simulink model "aerotest"  (R2021b)
settings: Solver=VariableStepAuto  StartTime=0.0  StopTime=10.0  RelTol=1e-3
undefined symbols (not defined in the file or in its folder): admireDB
libraries: simulink_extras x103, simulink x24, aerolibatmos2 x1
(part 9 of 13)

== system aerotest/CentripetalForceCoefficient/MachRegion4/Ccblg/Ccblg_ ==
  ldg : Inport
  angleOfAttack_deg : Inport  Port=2
  angleOfSideslip_deg : Inport  Port=3
  CCBLST_NG_DOOR_ALFA : Lookup_n-D  BreakpointsForDimension1=admireDB.aerodata_asym_ext.CCBLST.breakpoints.ALFA  BreakpointsForDimension2=admireDB.aerodata_asym_ext.CCBLST.breakpoints.NG_DOOR  BreakpointsForDimension3=[5, 7]  Table=admireDB.aerodata_asym_ext.CCBLST.newTable  ExtrapMethod=Clip  InternalRulePriority=Speed  RndMeth=Simplest  InputSameDT=on
      settings: InputPortMap=u0,u1
  Degrees to Radians : simulink_extras/Transformations/Degrees to Radians
  Product : Product  Inputs=3
  Ccblg : Outport
  wires:
  Degrees to Radians/1 -> Product/3
  CCBLST_NG_DOOR_ALFA/1 -> Product/2
  angleOfSideslip_deg/1 -> Degrees to Radians/1
  ldg/1 -> CCBLST_NG_DOOR_ALFA/2, Product/1
  angleOfAttack_deg/1 -> CCBLST_NG_DOOR_ALFA/1
  Product/1 -> Ccblg/1

== system aerotest/CentripetalForceCoefficient/MachRegion4/Ccdai/Ccdai_ ==
  dAI : Inport
  angleOfAttack_deg : Inport  Port=2
  dEI : Inport  Port=3
  qacorr : Inport  Port=4
  eieff : Inport  Port=5
  mach_nd : Inport  Port=6
  CCDA_ALFA_DE_M : Lookup_n-D  NumberOfTableDimensions=3  BreakpointsForDimension1=admireDB.aerodata_asym_ext.CCDA.breakpoints.ALFA  BreakpointsForDimension2=admireDB.aerodata_asym_ext.CCDA.breakpoints.DE  BreakpointsForDimension3=admireDB.aerodata_asym_ext.CCDA.breakpoints.M  Table=admireDB.aerodata_asym_ext.CCDA.newTable  ExtrapMethod=Clip  InternalRulePriority=Speed  RndMeth=Simplest  InputSameDT=on
      settings: InputPortMap=u0,u1,u2
  CCEDAI_QA_M : Lookup_n-D  BreakpointsForDimension1=admireDB.aerodata_asym_ext.CCEDAI.breakpoints.M  BreakpointsForDimension2=admireDB.aerodata_asym_ext.CCEDAI.breakpoints.QA  BreakpointsForDimension3=[5, 7]  Table=admireDB.aerodata_asym_ext.CCEDAI.newTable  ExtrapMethod=Clip  InternalRulePriority=Speed  RndMeth=Simplest  InputSameDT=on
      settings: InputPortMap=u0,u1
  Degrees to Radians : simulink_extras/Transformations/Degrees to Radians
  Product1 : Product  Inputs=4
  Ccdai : Outport
  wires:
  Product1/1 -> Ccdai/1
  eieff/1 -> Product1/2
  CCEDAI_QA_M/1 -> Product1/4
  qacorr/1 -> CCEDAI_QA_M/2
  dEI/1 -> CCDA_ALFA_DE_M/2
  CCDA_ALFA_DE_M/1 -> Product1/3
  Degrees to Radians/1 -> Product1/1
  mach_nd/1 -> CCDA_ALFA_DE_M/3, CCEDAI_QA_M/1
  angleOfAttack_deg/1 -> CCDA_ALFA_DE_M/1
  dAI/1 -> Degrees to Radians/1

== system aerotest/CentripetalForceCoefficient/MachRegion4/Ccday/Ccday_ ==
  angleOfAttack_deg : Inport
  dEY : Inport  Port=2
  mach_nd : Inport  Port=3
  qacorr : Inport  Port=4
  eoeff : Inport  Port=5
  dAY : Inport  Port=6
  CCDA_ALFA_DE_M : Lookup_n-D  NumberOfTableDimensions=3  BreakpointsForDimension1=admireDB.aerodata_asym_ext.CCDA.breakpoints.ALFA  BreakpointsForDimension2=admireDB.aerodata_asym_ext.CCDA.breakpoints.DE  BreakpointsForDimension3=admireDB.aerodata_asym_ext.CCDA.breakpoints.M  Table=admireDB.aerodata_asym_ext.CCDA.newTable  ExtrapMethod=Clip  InternalRulePriority=Speed  RndMeth=Simplest  InputSameDT=on
      settings: InputPortMap=u0,u1,u2
  CCEDAY_QA_M : Lookup_n-D  BreakpointsForDimension1=admireDB.aerodata_asym_ext.CCEDAY.breakpoints.M  BreakpointsForDimension2=admireDB.aerodata_asym_ext.CCEDAY.breakpoints.QA  BreakpointsForDimension3=[5, 7]  Table=admireDB.aerodata_asym_ext.CCEDAY.newTable  ExtrapMethod=Clip  InternalRulePriority=Speed  RndMeth=Simplest  InputSameDT=on
      settings: InputPortMap=u0,u1
  Degrees to Radians : simulink_extras/Transformations/Degrees to Radians
  Product : Product
  Product1 : Product
  Sum : Sum  Inputs=|++
  Ccday : Outport
  wires:
  Product1/1 -> Ccday/1
  dAY/1 -> Degrees to Radians/1
  Degrees to Radians/1 -> Product1/2
  Sum/1 -> Product1/1
  qacorr/1 -> CCEDAY_QA_M/2
  CCEDAY_QA_M/1 -> Sum/2
  Product/1 -> Sum/1
  CCDA_ALFA_DE_M/1 -> Product/1
  eoeff/1 -> Product/2
  mach_nd/1 -> CCDA_ALFA_DE_M/3, CCEDAY_QA_M/1
  dEY/1 -> CCDA_ALFA_DE_M/2
  angleOfAttack_deg/1 -> CCDA_ALFA_DE_M/1

== system aerotest/CentripetalForceCoefficient/MachRegion4/Ccdna/Ccdna_ ==
  angleOfAttack_deg : Inport
  mach_nd : Inport  Port=2
  dNA : Inport  Port=3
  CCDNAAM_ALFA_M : Lookup_n-D  BreakpointsForDimension1=admireDB.aerodata_asym_ext.CCDNAAM.breakpoints.M  BreakpointsForDimension2=admireDB.aerodata_asym_ext.CCDNAAM.breakpoints.ALFA  BreakpointsForDimension3=[5, 7]  Table=admireDB.aerodata_asym_ext.CCDNAAM.newTable  ExtrapMethod=Clip  InternalRulePriority=Speed  RndMeth=Simplest  InputSameDT=on
      settings: InputPortMap=u0,u1
  Degrees to Radians : simulink_extras/Transformations/Degrees to Radians
  Product1 : Product
  Ccdna : Outport
  wires:
  Degrees to Radians/1 -> Product1/2
  dNA/1 -> Degrees to Radians/1
  Product1/1 -> Ccdna/1
  mach_nd/1 -> CCDNAAM_ALFA_M/1
  CCDNAAM_ALFA_M/1 -> Product1/1
  angleOfAttack_deg/1 -> CCDNAAM_ALFA_M/2

== system aerotest/CentripetalForceCoefficient/MachRegion4/Ccdr/Ccdr_ ==
  angleOfAttack_deg : Inport
  mach_nd : Inport  Port=2
  dR : Inport  Port=3
  qacorr : Inport  Port=4
  CCDRAM_ALFA_M : Lookup_n-D  BreakpointsForDimension1=admireDB.aerodata_asym_ext.CCDRAM.breakpoints.M  BreakpointsForDimension2=admireDB.aerodata_asym_ext.CCDRAM.breakpoints.ALFA  BreakpointsForDimension3=[5, 7]  Table=admireDB.aerodata_asym_ext.CCDRAM.newTable  ExtrapMethod=Clip  InternalRulePriority=Speed  RndMeth=Simplest  InputSameDT=on
      settings: InputPortMap=u0,u1
  CCEDR_QA_M : Lookup_n-D  BreakpointsForDimension1=admireDB.aerodata_asym_ext.CCEDR.breakpoints.M  BreakpointsForDimension2=admireDB.aerodata_asym_ext.CCEDR.breakpoints.QA  BreakpointsForDimension3=[5, 7]  Table=admireDB.aerodata_asym_ext.CCEDR.newTable  ExtrapMethod=Clip  InternalRulePriority=Speed  RndMeth=Simplest  InputSameDT=on
      settings: InputPortMap=u0,u1
  Degrees to Radians : simulink_extras/Transformations/Degrees to Radians
  Product1 : Product  Inputs=3
  Ccdr : Outport
  wires:
  CCEDR_QA_M/1 -> Product1/3
  Product1/1 -> Ccdr/1
  mach_nd/1 -> CCEDR_QA_M/1, CCDRAM_ALFA_M/1
  qacorr/1 -> CCEDR_QA_M/2
  Degrees to Radians/1 -> Product1/2
  CCDRAM_ALFA_M/1 -> Product1/1
  dR/1 -> Degrees to Radians/1
  angleOfAttack_deg/1 -> CCDRAM_ALFA_M/2

== system aerotest/CentripetalForceCoefficient/MachRegion4/Ccp/Ccp_ ==
  angleOfAttack_deg : Inport
  mach_nd : Inport  Port=2
  pc : Inport  Port=3
  CCPAM_ALFA_M : Lookup_n-D  BreakpointsForDimension1=admireDB.aerodata_asym_ext.CCPAM.breakpoints.M  BreakpointsForDimension2=admireDB.aerodata_asym_ext.CCPAM.breakpoints.ALFA  BreakpointsForDimension3=[5, 7]  Table=admireDB.aerodata_asym_ext.CCPAM.newTable  ExtrapMethod=Clip  InternalRulePriority=Speed  RndMeth=Simplest  InputSameDT=on
      settings: InputPortMap=u0,u1
  Product2 : Product
  Ccp : Outport
  wires:
  mach_nd/1 -> CCPAM_ALFA_M/1
  CCPAM_ALFA_M/1 -> Product2/1
  Product2/1 -> Ccp/1
  pc/1 -> Product2/2
  angleOfAttack_deg/1 -> CCPAM_ALFA_M/2

== system aerotest/CentripetalForceCoefficient/MachRegion4/Ccr/Ccr_ ==
  mach_nd : Inport
  qacorr : Inport  Port=2
  rc : Inport  Port=3
  CCER_M_QA : Lookup_n-D  BreakpointsForDimension1=admireDB.aerodata_asym_ext.CCER.breakpoints.QA  BreakpointsForDimension2=admireDB.aerodata_asym_ext.CCER.breakpoints.M  BreakpointsForDimension3=[5, 7]  Table=admireDB.aerodata_asym_ext.CCER.newTable  ExtrapMethod=Clip  InternalRulePriority=Speed  RndMeth=Simplest  InputSameDT=on
      settings: InputPortMap=u0,u1
  CCRM_M : Lookup_n-D  NumberOfTableDimensions=1  BreakpointsForDimension1=admireDB.aerodata_asym_ext.CCRM.breakpoints.M  BreakpointsForDimension3=[5, 7]  Table=admireDB.aerodata_asym_ext.CCRM.newTable  ExtrapMethod=Clip  InternalRulePriority=Speed  RndMeth=Simplest  InputSameDT=on
  Product2 : Product  Inputs=3
  Ccr : Outport
  wires:
  CCER_M_QA/1 -> Product2/3
  qacorr/1 -> CCER_M_QA/1
  rc/1 -> Product2/2
  mach_nd/1 -> CCRM_M/1, CCER_M_QA/2
  CCRM_M/1 -> Product2/1
  Product2/1 -> Ccr/1

== system aerotest/NormalForceCoefficient/MachRegion2/Cndei/Subsystem ==
  <dEI> : Inport
  <angleOfAttack_deg> : Inport  Port=2
  CNMDEA_ALFA_DE_M : Lookup_n-D  NumberOfTableDimensions=3  BreakpointsForDimension1=admireDB.aerodata_sym.CNMDEA.breakpoints.ALFA  BreakpointsForDimension2=admireDB.aerodata_sym.CNMDEA.breakpoints.DE  BreakpointsForDimension3=admireDB.aerodata_sym.CNMDEA.breakpoints.M  Table=admireDB.aerodata_sym.CNMDEA.newTable  ExtrapMethod=Clip  InternalRulePriority=Speed  RndMeth=Simplest  InputSameDT=on
      settings: InputPortMap=u0,u1,u2
  CNMDEA_ALFA_DE_M1 : Lookup_n-D  NumberOfTableDimensions=3  BreakpointsForDimension1=admireDB.aerodata_sym.CNMDEA.breakpoints.ALFA  BreakpointsForDimension2=admireDB.aerodata_sym.CNMDEA.breakpoints.DE  BreakpointsForDimension3=admireDB.aerodata_sym.CNMDEA.breakpoints.M  Table=admireDB.aerodata_sym.CNMDEA.newTable  ExtrapMethod=Clip  InternalRulePriority=Speed  RndMeth=Simplest  InputSameDT=on
      settings: InputPortMap=u0,u1,u2
  Constant1 : Constant  Value=0
  Sum1 : Sum  Inputs=|+-
  mach_nd_cnst : Constant  Value=0.5
  Out1 : Outport
  wires:
  Constant1/1 -> CNMDEA_ALFA_DE_M1/2
  <dEI>/1 -> CNMDEA_ALFA_DE_M/2
  CNMDEA_ALFA_DE_M/1 -> Sum1/1
  CNMDEA_ALFA_DE_M1/1 -> Sum1/2
  Sum1/1 -> Out1/1
  mach_nd_cnst/1 -> CNMDEA_ALFA_DE_M/3, CNMDEA_ALFA_DE_M1/3
  <angleOfAttack_deg>/1 -> CNMDEA_ALFA_DE_M/1, CNMDEA_ALFA_DE_M1/1

== system aerotest/NormalForceCoefficient/MachRegion2/Cndei/Subsystem1 ==
  <dEI> : Inport
  <angleOfAttack_deg> : Inport  Port=2
  CNDEAL_DE_ALFA : Lookup_n-D  BreakpointsForDimension1=admireDB.aerodata_sym.CNDEAL.breakpoints.ALFA  BreakpointsForDimension2=admireDB.aerodata_sym.CNDEAL.breakpoints.DE  BreakpointsForDimension3=[5, 7]  Table=admireDB.aerodata_sym.CNDEAL.newTable  ExtrapMethod=Clip  InternalRulePriority=Speed  RndMeth=Simplest  InputSameDT=on
      settings: InputPortMap=u0,u1
  CNDEAL_DE_ALFA1 : Lookup_n-D  BreakpointsForDimension1=admireDB.aerodata_sym.CNDEAL.breakpoints.ALFA  BreakpointsForDimension2=admireDB.aerodata_sym.CNDEAL.breakpoints.DE  BreakpointsForDimension3=[5, 7]  Table=admireDB.aerodata_sym.CNDEAL.newTable  ExtrapMethod=Clip  InternalRulePriority=Speed  RndMeth=Simplest  InputSameDT=on
      settings: InputPortMap=u0,u1
  Constant : Constant  Value=0
  Sum : Sum  Inputs=|+-
  Out1 : Outport
  wires:
  <dEI>/1 -> CNDEAL_DE_ALFA/2
  CNDEAL_DE_ALFA/1 -> Sum/1
  Constant/1 -> CNDEAL_DE_ALFA1/2
  CNDEAL_DE_ALFA1/1 -> Sum/2
  Sum/1 -> Out1/1
  <angleOfAttack_deg>/1 -> CNDEAL_DE_ALFA/1, CNDEAL_DE_ALFA1/1

== system aerotest/NormalForceCoefficient/MachRegion2/Cndey/Subsystem ==
  dEY : Inport
  <angleOfAttack_deg> : Inport  Port=2
  CNMDEA_ALFA_DE_M : Lookup_n-D  NumberOfTableDimensions=3  BreakpointsForDimension1=admireDB.aerodata_sym.CNMDEA.breakpoints.ALFA  BreakpointsForDimension2=admireDB.aerodata_sym.CNMDEA.breakpoints.DE  BreakpointsForDimension3=admireDB.aerodata_sym.CNMDEA.breakpoints.M  Table=admireDB.aerodata_sym.CNMDEA.newTable  ExtrapMethod=Clip  InternalRulePriority=Speed  RndMeth=Simplest  InputSameDT=on
      settings: InputPortMap=u0,u1,u2
  CNMDEA_ALFA_DE_M1 : Lookup_n-D  NumberOfTableDimensions=3  BreakpointsForDimension1=admireDB.aerodata_sym.CNMDEA.breakpoints.ALFA  BreakpointsForDimension2=admireDB.aerodata_sym.CNMDEA.breakpoints.DE  BreakpointsForDimension3=admireDB.aerodata_sym.CNMDEA.breakpoints.M  Table=admireDB.aerodata_sym.CNMDEA.newTable  ExtrapMethod=Clip  InternalRulePriority=Speed  RndMeth=Simplest  InputSameDT=on
      settings: InputPortMap=u0,u1,u2
  Constant1 : Constant  Value=0
  Sum1 : Sum  Inputs=|+-
  mach_nd_cnst : Constant  Value=0.5
  Out1 : Outport
  wires:
  <angleOfAttack_deg>/1 -> CNMDEA_ALFA_DE_M1/1, CNMDEA_ALFA_DE_M/1
  mach_nd_cnst/1 -> CNMDEA_ALFA_DE_M1/3, CNMDEA_ALFA_DE_M/3
  Sum1/1 -> Out1/1
  CNMDEA_ALFA_DE_M1/1 -> Sum1/2
  CNMDEA_ALFA_DE_M/1 -> Sum1/1
  dEY/1 -> CNMDEA_ALFA_DE_M/2
  Constant1/1 -> CNMDEA_ALFA_DE_M1/2

== system aerotest/NormalForceCoefficient/MachRegion2/Cndey/Subsystem1 ==
  dEY : Inport
  <angleOfAttack_deg> : Inport  Port=2
  CNDEAL_DE_ALFA : Lookup_n-D  BreakpointsForDimension1=admireDB.aerodata_sym.CNDEAL.breakpoints.ALFA  BreakpointsForDimension2=admireDB.aerodata_sym.CNDEAL.breakpoints.DE  BreakpointsForDimension3=[5, 7]  Table=admireDB.aerodata_sym.CNDEAL.newTable  ExtrapMethod=Clip  InternalRulePriority=Speed  RndMeth=Simplest  InputSameDT=on
      settings: InputPortMap=u0,u1
  CNDEAL_DE_ALFA1 : Lookup_n-D  BreakpointsForDimension1=admireDB.aerodata_sym.CNDEAL.breakpoints.ALFA  BreakpointsForDimension2=admireDB.aerodata_sym.CNDEAL.breakpoints.DE  BreakpointsForDimension3=[5, 7]  Table=admireDB.aerodata_sym.CNDEAL.newTable  ExtrapMethod=Clip  InternalRulePriority=Speed  RndMeth=Simplest  InputSameDT=on
      settings: InputPortMap=u0,u1
  Constant : Constant  Value=0
  Sum : Sum  Inputs=|+-
  Out1 : Outport
  wires:
  <angleOfAttack_deg>/1 -> CNDEAL_DE_ALFA/1, CNDEAL_DE_ALFA1/1
  Sum/1 -> Out1/1
  CNDEAL_DE_ALFA1/1 -> Sum/2
  Constant/1 -> CNDEAL_DE_ALFA1/2
  CNDEAL_DE_ALFA/1 -> Sum/1
  dEY/1 -> CNDEAL_DE_ALFA/2

== system aerotest/NormalForceCoefficient/MachRegion2/Cndn/Subsystem ==
  dN : Inport
  angleOfAttack_deg : Inport  Port=2
  tflow : Inport  Port=3
  CNDNAL_DN_ALFA : Lookup_n-D  BreakpointsForDimension1=admireDB.aerodata_sym.CNDNAL.breakpoints.ALFA  BreakpointsForDimension2=admireDB.aerodata_sym.CNDNAL.breakpoints.DN  BreakpointsForDimension3=[5, 7]  Table=admireDB.aerodata_sym.CNDNAL.newTable  ExtrapMethod=Clip  InternalRulePriority=Speed  RndMeth=Simplest  InputSameDT=on
      settings: InputPortMap=u0,u1
  Product1 : Product
  Out1 : Outport
  wires:
  dN/1 -> CNDNAL_DN_ALFA/2  "dN"
  tflow/1 -> Product1/2  "tflow"
  angleOfAttack_deg/1 -> CNDNAL_DN_ALFA/1  "angleOfAttack_deg"
  Product1/1 -> Out1/1
  CNDNAL_DN_ALFA/1 -> Product1/1

== system aerotest/NormalForceCoefficient/MachRegion2/Cndn/Subsystem1 ==
  <dN> : Inport
  <angleOfAttack_deg> : Inport  Port=2
  <tfhigh> : Inport  Port=3
  CNDNH_M_DN_ALFA : Lookup_n-D  NumberOfTableDimensions=3  BreakpointsForDimension1=admireDB.aerodata_sym.CNDNH.breakpoints.M  BreakpointsForDimension2=admireDB.aerodata_sym.CNDNH.breakpoints.DN  BreakpointsForDimension3=admireDB.aerodata_sym.CNDNH.breakpoints.ALFA  Table=admireDB.aerodata_sym.CNDNH.newTable  ExtrapMethod=Clip  InternalRulePriority=Speed  RndMeth=Simplest  InputSameDT=on
      settings: InputPortMap=u0,u1,u2
  Product1 : Product
  mach_nd_cnst : Constant  Value=0.5
  Out1 : Outport
  wires:
  <dN>/1 -> CNDNH_M_DN_ALFA/2
  <tfhigh>/1 -> Product1/2
  <angleOfAttack_deg>/1 -> CNDNH_M_DN_ALFA/3
  CNDNH_M_DN_ALFA/1 -> Product1/1
  mach_nd_cnst/1 -> CNDNH_M_DN_ALFA/1
  Product1/1 -> Out1/1

== system aerotest/NormalForceCoefficient/MachRegion2/Cnq/Subsystem ==
  <angleOfAttack_deg> : Inport
  <tflow> : Inport  Port=2
  <tfhigh> : Inport  Port=3
  Abs : Abs
  CNQAL_ALFA : Lookup_n-D  NumberOfTableDimensions=1  BreakpointsForDimension1=admireDB.aerodata_sym.CNQAL.breakpoints.ALFA  BreakpointsForDimension3=[5, 7]  Table=admireDB.aerodata_sym.CNQAL.newTable  ExtrapMethod=Clip  InternalRulePriority=Speed  RndMeth=Simplest  InputSameDT=on
  CNQAM_ALFA_M : Lookup_n-D  BreakpointsForDimension1=admireDB.aerodata_sym.CNQAM.breakpoints.M  BreakpointsForDimension2=admireDB.aerodata_sym.CNQAM.breakpoints.ALFA  BreakpointsForDimension3=[5, 7]  Table=admireDB.aerodata_sym.CNQAM.newTable  ExtrapMethod=Clip  InternalRulePriority=Speed  RndMeth=Simplest  InputSameDT=on
      settings: InputPortMap=u0,u1
  Product : Product
  Product1 : Product
  Sum : Sum  Inputs=|++
  mach_nd_cnst : Constant  Value=0.5
  Out1 : Outport
  wires:
  <tfhigh>/1 -> Product1/2
  <tflow>/1 -> Product/2
  Product/1 -> Sum/1
  Sum/1 -> Out1/1
  CNQAL_ALFA/1 -> Product/1
  mach_nd_cnst/1 -> CNQAM_ALFA_M/1
  <angleOfAttack_deg>/1 -> CNQAM_ALFA_M/2, Abs/1
  Abs/1 -> CNQAL_ALFA/1
  Product1/1 -> Sum/2
  CNQAM_ALFA_M/1 -> Product1/1

== system aerotest/NormalForceCoefficient/MachRegion3/Cndei/Subsystem ==
  <angleOfAttack_deg> : Inport
  <dEI> : Inport  Port=2
  <mach_nd> : Inport  Port=3
  <eieff> : Inport  Port=4
  CNMDEA_ALFA_DE_M : Lookup_n-D  NumberOfTableDimensions=3  BreakpointsForDimension1=admireDB.aerodata_sym.CNMDEA.breakpoints.ALFA  BreakpointsForDimension2=admireDB.aerodata_sym.CNMDEA.breakpoints.DE  BreakpointsForDimension3=admireDB.aerodata_sym.CNMDEA.breakpoints.M  Table=admireDB.aerodata_sym.CNMDEA.newTable  ExtrapMethod=Clip  InternalRulePriority=Speed  RndMeth=Simplest  InputSameDT=on
      settings: InputPortMap=u0,u1,u2
  CNMDEA_ALFA_DE_M1 : Lookup_n-D  NumberOfTableDimensions=3  BreakpointsForDimension1=admireDB.aerodata_sym.CNMDEA.breakpoints.ALFA  BreakpointsForDimension2=admireDB.aerodata_sym.CNMDEA.breakpoints.DE  BreakpointsForDimension3=admireDB.aerodata_sym.CNMDEA.breakpoints.M  Table=admireDB.aerodata_sym.CNMDEA.newTable  ExtrapMethod=Clip  InternalRulePriority=Speed  RndMeth=Simplest  InputSameDT=on
      settings: InputPortMap=u0,u1,u2
  Constant : Constant  Value=0
  Product : Product
  Sum : Sum  Inputs=|+-
  Out1 : Outport
  wires:
  <eieff>/1 -> Product/2
  Product/1 -> Out1/1
  CNMDEA_ALFA_DE_M/1 -> Sum/1
  Constant/1 -> CNMDEA_ALFA_DE_M1/2
  <mach_nd>/1 -> CNMDEA_ALFA_DE_M/3, CNMDEA_ALFA_DE_M1/3
  Sum/1 -> Product/1
  <dEI>/1 -> CNMDEA_ALFA_DE_M/2
  <angleOfAttack_deg>/1 -> CNMDEA_ALFA_DE_M/1, CNMDEA_ALFA_DE_M1/1
  CNMDEA_ALFA_DE_M1/1 -> Sum/2

== system aerotest/NormalForceCoefficient/MachRegion3/Cndey/Subsystem ==
  <angleOfAttack_deg> : Inport
  <dEI> : Inport  Port=2
  <mach_nd> : Inport  Port=3
  <eieff> : Inport  Port=4
  CNMDEA_ALFA_DE_M : Lookup_n-D  NumberOfTableDimensions=3  BreakpointsForDimension1=admireDB.aerodata_sym.CNMDEA.breakpoints.ALFA  BreakpointsForDimension2=admireDB.aerodata_sym.CNMDEA.breakpoints.DE  BreakpointsForDimension3=admireDB.aerodata_sym.CNMDEA.breakpoints.M  Table=admireDB.aerodata_sym.CNMDEA.newTable  ExtrapMethod=Clip  InternalRulePriority=Speed  RndMeth=Simplest  InputSameDT=on
      settings: InputPortMap=u0,u1,u2
  CNMDEA_ALFA_DE_M1 : Lookup_n-D  NumberOfTableDimensions=3  BreakpointsForDimension1=admireDB.aerodata_sym.CNMDEA.breakpoints.ALFA  BreakpointsForDimension2=admireDB.aerodata_sym.CNMDEA.breakpoints.DE  BreakpointsForDimension3=admireDB.aerodata_sym.CNMDEA.breakpoints.M  Table=admireDB.aerodata_sym.CNMDEA.newTable  ExtrapMethod=Clip  InternalRulePriority=Speed  RndMeth=Simplest  InputSameDT=on
      settings: InputPortMap=u0,u1,u2
  Constant : Constant  Value=0
  Product : Product
  Sum : Sum  Inputs=|+-
  Out1 : Outport
  wires:
  CNMDEA_ALFA_DE_M1/1 -> Sum/2
  <angleOfAttack_deg>/1 -> CNMDEA_ALFA_DE_M1/1, CNMDEA_ALFA_DE_M/1
  <dEI>/1 -> CNMDEA_ALFA_DE_M/2
  Sum/1 -> Product/1
  <mach_nd>/1 -> CNMDEA_ALFA_DE_M1/3, CNMDEA_ALFA_DE_M/3
  Constant/1 -> CNMDEA_ALFA_DE_M1/2
  CNMDEA_ALFA_DE_M/1 -> Sum/1
  Product/1 -> Out1/1
  <eieff>/1 -> Product/2

== system aerotest/PitchMomentCoefficient/MachRegion1/Cpmdei/Subsystem ==
  <dEI> : Inport
  <angleOfAttack_deg> : Inport  Port=2
  <eieff> : Inport  Port=3
  CPMDEAL_DE_ALFA1 : Lookup_n-D  BreakpointsForDimension1=admireDB.aerodata_sym.CPMDEAL.breakpoints.ALFA  BreakpointsForDimension2=admireDB.aerodata_sym.CPMDEAL.breakpoints.DE  BreakpointsForDimension3=[5, 7]  Table=admireDB.aerodata_sym.CPMDEAL.newTable  ExtrapMethod=Clip  InternalRulePriority=Speed  RndMeth=Simplest  InputSameDT=on
      settings: InputPortMap=u0,u1
  CPMDEAL_DE_ALFA2 : Lookup_n-D  BreakpointsForDimension1=admireDB.aerodata_sym.CPMDEAL.breakpoints.ALFA  BreakpointsForDimension2=admireDB.aerodata_sym.CPMDEAL.breakpoints.DE  BreakpointsForDimension3=[5, 7]  Table=admireDB.aerodata_sym.CPMDEAL.newTable  ExtrapMethod=Clip  InternalRulePriority=Speed  RndMeth=Simplest  InputSameDT=on
      settings: InputPortMap=u0,u1
  Constant : Constant  Value=0
  Product : Product
  Sum : Sum  Inputs=|+-
  Out1 : Outport
  wires:
  <dEI>/1 -> CPMDEAL_DE_ALFA1/2
  Product/1 -> Out1/1
  CPMDEAL_DE_ALFA1/1 -> Sum/1
  CPMDEAL_DE_ALFA2/1 -> Sum/2
  Sum/1 -> Product/1
  <angleOfAttack_deg>/1 -> CPMDEAL_DE_ALFA1/1, CPMDEAL_DE_ALFA2/1
  Constant/1 -> CPMDEAL_DE_ALFA2/2
  <eieff>/1 -> Product/2

== system aerotest/PitchMomentCoefficient/MachRegion1/Cpmdey/Subsystem ==
  dEY : Inport
  angleOfAttack_deg : Inport  Port=2
  eoeff : Inport  Port=3
  CPMDEAL_DE_ALFA1 : Lookup_n-D  BreakpointsForDimension1=admireDB.aerodata_sym.CPMDEAL.breakpoints.ALFA  BreakpointsForDimension2=admireDB.aerodata_sym.CPMDEAL.breakpoints.DE  BreakpointsForDimension3=[5, 7]  Table=admireDB.aerodata_sym.CPMDEAL.newTable  ExtrapMethod=Clip  InternalRulePriority=Speed  RndMeth=Simplest  InputSameDT=on
      settings: InputPortMap=u0,u1
  CPMDEAL_DE_ALFA2 : Lookup_n-D  BreakpointsForDimension1=admireDB.aerodata_sym.CPMDEAL.breakpoints.ALFA  BreakpointsForDimension2=admireDB.aerodata_sym.CPMDEAL.breakpoints.DE  BreakpointsForDimension3=[5, 7]  Table=admireDB.aerodata_sym.CPMDEAL.newTable  ExtrapMethod=Clip  InternalRulePriority=Speed  RndMeth=Simplest  InputSameDT=on
      settings: InputPortMap=u0,u1
  Constant : Constant  Value=0
  Product : Product
  Sum : Sum  Inputs=|+-
  Out1 : Outport
  wires:
  eoeff/1 -> Product/2
  Constant/1 -> CPMDEAL_DE_ALFA2/2
  angleOfAttack_deg/1 -> CPMDEAL_DE_ALFA2/1, CPMDEAL_DE_ALFA1/1
  Sum/1 -> Product/1
  CPMDEAL_DE_ALFA2/1 -> Sum/2
  CPMDEAL_DE_ALFA1/1 -> Sum/1
  Product/1 -> Out1/1
  dEY/1 -> CPMDEAL_DE_ALFA1/2

== system aerotest/PitchMomentCoefficient/MachRegion1/Cpmdle/Subsystem ==
  <angleOfAttack_deg> : Inport
  <dE> : Inport  Port=2
  <dN> : Inport  Port=3
  <lef_deg> : Inport  Port=4
  CPMDLAL_ALFA : Lookup_n-D  NumberOfTableDimensions=1  BreakpointsForDimension1=admireDB.aerodata_sym.CPMDLAL.breakpoints.ALFA  BreakpointsForDimension3=[5, 7]  Table=admireDB.aerodata_sym.CPMDLAL.newTable  ExtrapMethod=Clip  InternalRulePriority=Speed  RndMeth=Simplest  InputSameDT=on
  CPMDLDEA_DE_ALFA : Lookup_n-D  BreakpointsForDimension1=admireDB.aerodata_sym.CPMDLDEA.breakpoints.ALFA  BreakpointsForDimension2=admireDB.aerodata_sym.CPMDLDEA.breakpoints.DE  BreakpointsForDimension3=[5, 7]  Table=admireDB.aerodata_sym.CPMDLDEA.newTable  ExtrapMethod=Clip  InternalRulePriority=Speed  RndMeth=Simplest  InputSameDT=on
      settings: InputPortMap=u0,u1
  CPMDLDNA_DN_ALFA : Lookup_n-D  BreakpointsForDimension1=admireDB.aerodata_sym.CPMDLDNA.breakpoints.ALFA  BreakpointsForDimension2=admireDB.aerodata_sym.CPMDLDNA.breakpoints.DN  BreakpointsForDimension3=[5, 7]  Table=admireDB.aerodata_sym.CPMDLDNA.newTable  ExtrapMethod=Clip  InternalRulePriority=Speed  RndMeth=Simplest  InputSameDT=on
      settings: InputPortMap=u0,u1
  Constant : Constant  Value=1/27
  Product : Product  Inputs=3
  Sum : Sum  Inputs=+++
  Out1 : Outport
  wires:
  Constant/1 -> Product/3
  <lef_deg>/1 -> Product/2
  <dN>/1 -> CPMDLDNA_DN_ALFA/2
  Product/1 -> Out1/1
  CPMDLDEA_DE_ALFA/1 -> Sum/2
  <angleOfAttack_deg>/1 -> CPMDLDNA_DN_ALFA/1, CPMDLDEA_DE_ALFA/1, CPMDLAL_ALFA/1
  CPMDLAL_ALFA/1 -> Sum/1
  Sum/1 -> Product/1
  CPMDLDNA_DN_ALFA/1 -> Sum/3
  <dE>/1 -> CPMDLDEA_DE_ALFA/2

== system aerotest/PitchMomentCoefficient/MachRegion1/Cpmdle/Subsystem1 ==
  <qacorr> : Inport
  <mach_nd> : Inport  Port=2
  CPMEDLEI_QA_M : Lookup_n-D  BreakpointsForDimension1=admireDB.aerodata_sym.CPMEDLEI.breakpoints.M  BreakpointsForDimension2=admireDB.aerodata_sym.CPMEDLEI.breakpoints.QA  BreakpointsForDimension3=[5, 7]  Table=admireDB.aerodata_sym.CPMEDLEI.newTable  ExtrapMethod=Clip  InternalRulePriority=Speed  RndMeth=Simplest  InputSameDT=on
      settings: InputPortMap=u0,u1
  CPMEDLEY_QA_M : Lookup_n-D  BreakpointsForDimension1=admireDB.aerodata_sym.CPMEDLEY.breakpoints.M  BreakpointsForDimension2=admireDB.aerodata_sym.CPMEDLEY.breakpoints.QA  BreakpointsForDimension3=[5, 7]  Table=admireDB.aerodata_sym.CPMEDLEY.newTable  ExtrapMethod=Clip  InternalRulePriority=Speed  RndMeth=Simplest  InputSameDT=on
      settings: InputPortMap=u0,u1
  Sum1 : Sum  Inputs=|++
  Out1 : Outport
  wires:
  Sum1/1 -> Out1/1
  <mach_nd>/1 -> CPMEDLEI_QA_M/1, CPMEDLEY_QA_M/1
  CPMEDLEI_QA_M/1 -> Sum1/1
  CPMEDLEY_QA_M/1 -> Sum1/2
  <qacorr>/1 -> CPMEDLEY_QA_M/2, CPMEDLEI_QA_M/2

== system aerotest/PitchMomentCoefficient/MachRegion2/Cpmalfa/CPMDEAL ==
  angleOfAttack_deg : Inport
  tflow : Inport  Port=2
  CPMDEAL_DE_ALFA : Lookup_n-D  BreakpointsForDimension1=admireDB.aerodata_sym.CPMDEAL.breakpoints.ALFA  BreakpointsForDimension2=admireDB.aerodata_sym.CPMDEAL.breakpoints.DE  BreakpointsForDimension3=[5, 7]  Table=admireDB.aerodata_sym.CPMDEAL.newTable  ExtrapMethod=Clip  InternalRulePriority=Speed  RndMeth=Simplest  InputSameDT=on
      settings: InputPortMap=u0,u1
  Product1 : Product
  dE_cnst : Constant  Value=0.0
  Out1 : Outport
  wires:
  tflow/1 -> Product1/2
  Product1/1 -> Out1/1
  CPMDEAL_DE_ALFA/1 -> Product1/1
  dE_cnst/1 -> CPMDEAL_DE_ALFA/2
  angleOfAttack_deg/1 -> CPMDEAL_DE_ALFA/1

== system aerotest/PitchMomentCoefficient/MachRegion2/Cpmalfa/CPMMDEA ==
  tfhigh : Inport
  angleOfAttack_deg : Inport  Port=2
  CPMMDEA_ALFA_DE_M : Lookup_n-D  NumberOfTableDimensions=3  BreakpointsForDimension1=admireDB.aerodata_sym.CPMMDEA.breakpoints.ALFA  BreakpointsForDimension2=admireDB.aerodata_sym.CPMMDEA.breakpoints.DE  BreakpointsForDimension3=admireDB.aerodata_sym.CPMMDEA.breakpoints.M  Table=admireDB.aerodata_sym.CPMMDEA.newTable  ExtrapMethod=Clip  InternalRulePriority=Speed  RndMeth=Simplest  InputSameDT=on
      settings: InputPortMap=u0,u1,u2
  Product2 : Product
  dE_cnst1 : Constant  Value=0.0
  mach_nd_cnst : Constant  Value=0.5
  Out1 : Outport
  wires:
  Product2/1 -> Out1/1
  CPMMDEA_ALFA_DE_M/1 -> Product2/2
  tfhigh/1 -> Product2/1
  mach_nd_cnst/1 -> CPMMDEA_ALFA_DE_M/3
  angleOfAttack_deg/1 -> CPMMDEA_ALFA_DE_M/1
  dE_cnst1/1 -> CPMMDEA_ALFA_DE_M/2

== system aerotest/PitchMomentCoefficient/MachRegion2/Cpmda/CPMDAAL ==
  dAI : Inport
  angleOfAttack_deg : Inport  Port=2
  eiefflow : Inport  Port=3
  dAY : Inport  Port=4
  eoefflow : Inport  Port=5
  Abs : Abs
  Abs1 : Abs
  CPMDAAL_DA_ALFA : Lookup_n-D  BreakpointsForDimension1=admireDB.aerodata_sym.CPMDAAL.breakpoints.ALFA  BreakpointsForDimension2=admireDB.aerodata_sym.CPMDAAL.breakpoints.DA  BreakpointsForDimension3=[5, 7]  Table=admireDB.aerodata_sym.CPMDAAL.newTable  ExtrapMethod=Clip  InternalRulePriority=Speed  RndMeth=Simplest  InputSameDT=on
      settings: InputPortMap=u0,u1
  CPMDAAL_DA_ALFA1 : Lookup_n-D  BreakpointsForDimension1=admireDB.aerodata_sym.CPMDAAL.breakpoints.ALFA  BreakpointsForDimension2=admireDB.aerodata_sym.CPMDAAL.breakpoints.DA  BreakpointsForDimension3=[5, 7]  Table=admireDB.aerodata_sym.CPMDAAL.newTable  ExtrapMethod=Clip  InternalRulePriority=Speed  RndMeth=Simplest  InputSameDT=on
      settings: InputPortMap=u0,u1
  Product : Product
  Product1 : Product
  Sum : Sum  Inputs=|++
  Out1 : Outport
  wires:
  eoefflow/1 -> Product1/2
  dAY/1 -> Abs1/1
  eiefflow/1 -> Product/2
  dAI/1 -> Abs/1
  Product1/1 -> Sum/2
  CPMDAAL_DA_ALFA/1 -> Product/1
  Abs1/1 -> CPMDAAL_DA_ALFA1/2
  CPMDAAL_DA_ALFA1/1 -> Product1/1
  Sum/1 -> Out1/1
  Abs/1 -> CPMDAAL_DA_ALFA/2
  Product/1 -> Sum/1
  angleOfAttack_deg/1 -> CPMDAAL_DA_ALFA/1, CPMDAAL_DA_ALFA1/1

== system aerotest/PitchMomentCoefficient/MachRegion2/Cpmdei/CPMDEAL ==
  dEI : Inport
  angleOfAttack_deg : Inport  Port=2
  tflow : Inport  Port=3
  CPMDEAL_DE_ALFA1 : Lookup_n-D  BreakpointsForDimension1=admireDB.aerodata_sym.CPMDEAL.breakpoints.ALFA  BreakpointsForDimension2=admireDB.aerodata_sym.CPMDEAL.breakpoints.DE  BreakpointsForDimension3=[5, 7]  Table=admireDB.aerodata_sym.CPMDEAL.newTable  ExtrapMethod=Clip  InternalRulePriority=Speed  RndMeth=Simplest  InputSameDT=on
      settings: InputPortMap=u0,u1
  CPMDEAL_DE_ALFA2 : Lookup_n-D  BreakpointsForDimension1=admireDB.aerodata_sym.CPMDEAL.breakpoints.ALFA  BreakpointsForDimension2=admireDB.aerodata_sym.CPMDEAL.breakpoints.DE  BreakpointsForDimension3=[5, 7]  Table=admireDB.aerodata_sym.CPMDEAL.newTable  ExtrapMethod=Clip  InternalRulePriority=Speed  RndMeth=Simplest  InputSameDT=on
      settings: InputPortMap=u0,u1
  Constant : Constant  Value=0
  Product : Product
  Sum : Sum  Inputs=|+-
  Out1 : Outport
  wires:
  tflow/1 -> Product/2
  Constant/1 -> CPMDEAL_DE_ALFA2/2
  angleOfAttack_deg/1 -> CPMDEAL_DE_ALFA1/1, CPMDEAL_DE_ALFA2/1
  Sum/1 -> Product/1
  CPMDEAL_DE_ALFA2/1 -> Sum/2
  CPMDEAL_DE_ALFA1/1 -> Sum/1
  Product/1 -> Out1/1
  dEI/1 -> CPMDEAL_DE_ALFA1/2

== system aerotest/PitchMomentCoefficient/MachRegion2/Cpmdei/CPMMDEA ==
  tfhigh : Inport
  angleOfAttack_deg : Inport  Port=2
  dEI : Inport  Port=3
  CPMMDEA_ALFA_DE_M : Lookup_n-D  NumberOfTableDimensions=3  BreakpointsForDimension1=admireDB.aerodata_sym.CPMMDEA.breakpoints.ALFA  BreakpointsForDimension2=admireDB.aerodata_sym.CPMMDEA.breakpoints.DE  BreakpointsForDimension3=admireDB.aerodata_sym.CPMMDEA.breakpoints.M  Table=admireDB.aerodata_sym.CPMMDEA.newTable  ExtrapMethod=Clip  InternalRulePriority=Speed  RndMeth=Simplest  InputSameDT=on
      settings: InputPortMap=u0,u1,u2
  CPMMDEA_ALFA_DE_M1 : Lookup_n-D  NumberOfTableDimensions=3  BreakpointsForDimension1=admireDB.aerodata_sym.CPMMDEA.breakpoints.ALFA  BreakpointsForDimension2=admireDB.aerodata_sym.CPMMDEA.breakpoints.DE  BreakpointsForDimension3=admireDB.aerodata_sym.CPMMDEA.breakpoints.M  Table=admireDB.aerodata_sym.CPMMDEA.newTable  ExtrapMethod=Clip  InternalRulePriority=Speed  RndMeth=Simplest  InputSameDT=on
      settings: InputPortMap=u0,u1,u2
  Constant1 : Constant  Value=0.5
  Constant2 : Constant  Value=0
  Product : Product
  Sum : Sum  Inputs=|+-
  Out1 : Outport
  wires:
  CPMMDEA_ALFA_DE_M1/1 -> Sum/2
  Constant2/1 -> CPMMDEA_ALFA_DE_M1/2
  Constant1/1 -> CPMMDEA_ALFA_DE_M1/3, CPMMDEA_ALFA_DE_M/3
  dEI/1 -> CPMMDEA_ALFA_DE_M/2
  Product/1 -> Out1/1
  CPMMDEA_ALFA_DE_M/1 -> Sum/1
  Sum/1 -> Product/1
  angleOfAttack_deg/1 -> CPMMDEA_ALFA_DE_M/1, CPMMDEA_ALFA_DE_M1/1
  tfhigh/1 -> Product/2

== system aerotest/PitchMomentCoefficient/MachRegion2/Cpmdey/CPMDEAL ==
  dEI : Inport
  angleOfAttack_deg : Inport  Port=2
  tflow : Inport  Port=3
  CPMDEAL_DE_ALFA1 : Lookup_n-D  BreakpointsForDimension1=admireDB.aerodata_sym.CPMDEAL.breakpoints.ALFA  BreakpointsForDimension2=admireDB.aerodata_sym.CPMDEAL.breakpoints.DE  BreakpointsForDimension3=[5, 7]  Table=admireDB.aerodata_sym.CPMDEAL.newTable  ExtrapMethod=Clip  InternalRulePriority=Speed  RndMeth=Simplest  InputSameDT=on
      settings: InputPortMap=u0,u1
  CPMDEAL_DE_ALFA2 : Lookup_n-D  BreakpointsForDimension1=admireDB.aerodata_sym.CPMDEAL.breakpoints.ALFA  BreakpointsForDimension2=admireDB.aerodata_sym.CPMDEAL.breakpoints.DE  BreakpointsForDimension3=[5, 7]  Table=admireDB.aerodata_sym.CPMDEAL.newTable  ExtrapMethod=Clip  InternalRulePriority=Speed  RndMeth=Simplest  InputSameDT=on
      settings: InputPortMap=u0,u1
  Constant : Constant  Value=0
  Product : Product
  Sum : Sum  Inputs=|+-
  Out1 : Outport
  wires:
  Constant/1 -> CPMDEAL_DE_ALFA2/2
  dEI/1 -> CPMDEAL_DE_ALFA1/2
  Product/1 -> Out1/1
  CPMDEAL_DE_ALFA1/1 -> Sum/1
  CPMDEAL_DE_ALFA2/1 -> Sum/2
  Sum/1 -> Product/1
  angleOfAttack_deg/1 -> CPMDEAL_DE_ALFA1/1, CPMDEAL_DE_ALFA2/1
  tflow/1 -> Product/2

== system aerotest/PitchMomentCoefficient/MachRegion2/Cpmdey/CPMMDEA ==
  tfhigh : Inport
  angleOfAttack_deg : Inport  Port=2
  dEI : Inport  Port=3
  CPMMDEA_ALFA_DE_M : Lookup_n-D  NumberOfTableDimensions=3  BreakpointsForDimension1=admireDB.aerodata_sym.CPMMDEA.breakpoints.ALFA  BreakpointsForDimension2=admireDB.aerodata_sym.CPMMDEA.breakpoints.DE  BreakpointsForDimension3=admireDB.aerodata_sym.CPMMDEA.breakpoints.M  Table=admireDB.aerodata_sym.CPMMDEA.newTable  ExtrapMethod=Clip  InternalRulePriority=Speed  RndMeth=Simplest  InputSameDT=on
      settings: InputPortMap=u0,u1,u2
  CPMMDEA_ALFA_DE_M1 : Lookup_n-D  NumberOfTableDimensions=3  BreakpointsForDimension1=admireDB.aerodata_sym.CPMMDEA.breakpoints.ALFA  BreakpointsForDimension2=admireDB.aerodata_sym.CPMMDEA.breakpoints.DE  BreakpointsForDimension3=admireDB.aerodata_sym.CPMMDEA.breakpoints.M  Table=admireDB.aerodata_sym.CPMMDEA.newTable  ExtrapMethod=Clip  InternalRulePriority=Speed  RndMeth=Simplest  InputSameDT=on
      settings: InputPortMap=u0,u1,u2
  Constant1 : Constant  Value=0.5
  Constant2 : Constant  Value=0
  Product : Product
  Sum : Sum  Inputs=|+-
  Out1 : Outport
  wires:
  tfhigh/1 -> Product/2
  angleOfAttack_deg/1 -> CPMMDEA_ALFA_DE_M1/1, CPMMDEA_ALFA_DE_M/1
  Sum/1 -> Product/1
  CPMMDEA_ALFA_DE_M/1 -> Sum/1
  Product/1 -> Out1/1
  dEI/1 -> CPMMDEA_ALFA_DE_M/2
  Constant1/1 -> CPMMDEA_ALFA_DE_M/3, CPMMDEA_ALFA_DE_M1/3
  Constant2/1 -> CPMMDEA_ALFA_DE_M1/2
  CPMMDEA_ALFA_DE_M1/1 -> Sum/2

== system aerotest/PitchMomentCoefficient/MachRegion2/Cpmdle/Subsystem ==
  angleOfAttack_deg : Inport
  dE : Inport  Port=2
  dN : Inport  Port=3
  tflow : Inport  Port=4
  tfhigh : Inport  Port=5
  lef_deg : Inport  Port=6
  " mach_nd_cnst" : Constant  Value=0.5
  CPMDLAL_ALFA : Lookup_n-D  NumberOfTableDimensions=1  BreakpointsForDimension1=admireDB.aerodata_sym.CPMDLAL.breakpoints.ALFA  BreakpointsForDimension3=[5, 7]  Table=admireDB.aerodata_sym.CPMDLAL.newTable  ExtrapMethod=Clip  InternalRulePriority=Speed  RndMeth=Simplest  InputSameDT=on
  CPMDLDEA_DE_ALFA : Lookup_n-D  BreakpointsForDimension1=admireDB.aerodata_sym.CPMDLDEA.breakpoints.ALFA  BreakpointsForDimension2=admireDB.aerodata_sym.CPMDLDEA.breakpoints.DE  BreakpointsForDimension3=[5, 7]  Table=admireDB.aerodata_sym.CPMDLDEA.newTable  ExtrapMethod=Clip  InternalRulePriority=Speed  RndMeth=Simplest  InputSameDT=on
      settings: InputPortMap=u0,u1
  CPMDLDNA_DN_ALFA : Lookup_n-D  BreakpointsForDimension1=admireDB.aerodata_sym.CPMDLDNA.breakpoints.ALFA  BreakpointsForDimension2=admireDB.aerodata_sym.CPMDLDNA.breakpoints.DN  BreakpointsForDimension3=[5, 7]  Table=admireDB.aerodata_sym.CPMDLDNA.newTable  ExtrapMethod=Clip  InternalRulePriority=Speed  RndMeth=Simplest  InputSameDT=on
      settings: InputPortMap=u0,u1
  CPMMDLEA_ALFA_DLE_M : Lookup_n-D  NumberOfTableDimensions=3  BreakpointsForDimension1=admireDB.aerodata_sym.CPMMDLEA.breakpoints.ALFA  BreakpointsForDimension2=admireDB.aerodata_sym.CPMMDLEA.breakpoints.DLE  BreakpointsForDimension3=admireDB.aerodata_sym.CPMMDLEA.breakpoints.M  Table=admireDB.aerodata_sym.CPMMDLEA.newTable  ExtrapMethod=Clip  InternalRulePriority=Speed  RndMeth=Simplest  InputSameDT=on
      settings: InputPortMap=u0,u1,u2
  Constant : Constant  Value=1/27
  Product : Product  Inputs=4
  Product1 : Product
  Sum : Sum  Inputs=+++
  Sum1 : Sum  Inputs=|++
  Out1 : Outport
  wires:
  Product1/1 -> Sum1/2
  Sum1/1 -> Out1/1
  tfhigh/1 -> Product1/1
  CPMMDLEA_ALFA_DLE_M/1 -> Product1/2
  angleOfAttack_deg/1 -> CPMDLAL_ALFA/1, CPMDLDEA_DE_ALFA/1, CPMDLDNA_DN_ALFA/1, CPMMDLEA_ALFA_DLE_M/1
  lef_deg/1 -> Product/3, CPMMDLEA_ALFA_DLE_M/2
  " mach_nd_cnst"/1 -> CPMMDLEA_ALFA_DLE_M/3
  tflow/1 -> Product/1
  dE/1 -> CPMDLDEA_DE_ALFA/2
  CPMDLDNA_DN_ALFA/1 -> Sum/3
  Sum/1 -> Product/2
  CPMDLAL_ALFA/1 -> Sum/1
  CPMDLDEA_DE_ALFA/1 -> Sum/2
  Product/1 -> Sum1/1
  dN/1 -> CPMDLDNA_DN_ALFA/2
  Constant/1 -> Product/4

== system aerotest/PitchMomentCoefficient/MachRegion2/Cpmdle/Subsystem1 ==
  qacorr : Inport
  mach_nd : Inport  Port=2
  CPMEDLEI_QA_M : Lookup_n-D  BreakpointsForDimension1=admireDB.aerodata_sym.CPMEDLEI.breakpoints.M  BreakpointsForDimension2=admireDB.aerodata_sym.CPMEDLEI.breakpoints.QA  BreakpointsForDimension3=[5, 7]  Table=admireDB.aerodata_sym.CPMEDLEI.newTable  ExtrapMethod=Clip  InternalRulePriority=Speed  RndMeth=Simplest  InputSameDT=on
      settings: InputPortMap=u0,u1
  CPMEDLEY_QA_M : Lookup_n-D  BreakpointsForDimension1=admireDB.aerodata_sym.CPMEDLEY.breakpoints.M  BreakpointsForDimension2=admireDB.aerodata_sym.CPMEDLEY.breakpoints.QA  BreakpointsForDimension3=[5, 7]  Table=admireDB.aerodata_sym.CPMEDLEY.newTable  ExtrapMethod=Clip  InternalRulePriority=Speed  RndMeth=Simplest  InputSameDT=on
      settings: InputPortMap=u0,u1
  Sum1 : Sum  Inputs=|++
  Out1 : Outport
  wires:
  mach_nd/1 -> CPMEDLEY_QA_M/1, CPMEDLEI_QA_M/1
  CPMEDLEY_QA_M/1 -> Sum1/2
  CPMEDLEI_QA_M/1 -> Sum1/1
  qacorr/1 -> CPMEDLEY_QA_M/2, CPMEDLEI_QA_M/2
  Sum1/1 -> Out1/1

== system aerotest/PitchMomentCoefficient/MachRegion2/Cpmdn/CPMDNAL_CPMMDNA ==
  dN : Inport
  angleOfAttack_deg : Inport  Port=2
  tflow : Inport  Port=3
  tfhigh : Inport  Port=4
  CPMDNAL_DN_ALFA : Lookup_n-D  BreakpointsForDimension1=admireDB.aerodata_sym.CPMDNAL.breakpoints.ALFA  BreakpointsForDimension2=admireDB.aerodata_sym.CPMDNAL.breakpoints.DN  BreakpointsForDimension3=[5, 7]  Table=admireDB.aerodata_sym.CPMDNAL.newTable  ExtrapMethod=Clip  InternalRulePriority=Speed  RndMeth=Simplest  InputSameDT=on
      settings: InputPortMap=u0,u1
  CPMMDNA_ALFA_DN_M : Lookup_n-D  NumberOfTableDimensions=3  BreakpointsForDimension1=admireDB.aerodata_sym.CPMMDNA.breakpoints.ALFA  BreakpointsForDimension2=admireDB.aerodata_sym.CPMMDNA.breakpoints.DN  BreakpointsForDimension3=admireDB.aerodata_sym.CPMMDNA.breakpoints.M  Table=admireDB.aerodata_sym.CPMMDNA.newTable  ExtrapMethod=Clip  InternalRulePriority=Speed  RndMeth=Simplest  InputSameDT=on
      settings: InputPortMap=u0,u1,u2
  Product : Product
  Product1 : Product
  Sum : Sum  Inputs=|++
  mach_nd_cnst : Constant  Value=0.5
  Out1 : Outport
  wires:
  Product1/1 -> Sum/2
  tfhigh/1 -> Product1/1
  Product/1 -> Sum/1
  tflow/1 -> Product/2
  mach_nd_cnst/1 -> CPMMDNA_ALFA_DN_M/3
  Sum/1 -> Out1/1
  angleOfAttack_deg/1 -> CPMDNAL_DN_ALFA/1, CPMMDNA_ALFA_DN_M/1
  CPMDNAL_DN_ALFA/1 -> Product/1
  dN/1 -> CPMDNAL_DN_ALFA/2, CPMMDNA_ALFA_DN_M/2
  CPMMDNA_ALFA_DN_M/1 -> Product1/2

== system aerotest/PitchMomentCoefficient/MachRegion2/Cpmq/Subsystem ==
  tflow : Inport
  angleOfAttack_deg : Inport  Port=2
  dN : Inport  Port=3
  tfhigh : Inport  Port=4
  CPMQAL_ALFA : Lookup_n-D  NumberOfTableDimensions=1  BreakpointsForDimension1=admireDB.aerodata_sym.CPMQAL.breakpoints.ALFA  BreakpointsForDimension3=[5, 7]  Table=admireDB.aerodata_sym.CPMQAL.newTable  ExtrapMethod=Clip  InternalRulePriority=Speed  RndMeth=Simplest  InputSameDT=on
  CPMQAM_ALFA_M : Lookup_n-D  BreakpointsForDimension1=admireDB.aerodata_sym.CPMQAM.breakpoints.M  BreakpointsForDimension2=admireDB.aerodata_sym.CPMQAM.breakpoints.ALFA  BreakpointsForDimension3=[5, 7]  Table=admireDB.aerodata_sym.CPMQAM.newTable  ExtrapMethod=Clip  InternalRulePriority=Speed  RndMeth=Simplest  InputSameDT=on
      settings: InputPortMap=u0,u1
  CPMQDNAL_DN_ALFA : Lookup_n-D  BreakpointsForDimension1=admireDB.aerodata_sym.CPMQDNAL.breakpoints.ALFA  BreakpointsForDimension2=admireDB.aerodata_sym.CPMQDNAL.breakpoints.DN  BreakpointsForDimension3=[5, 7]  Table=admireDB.aerodata_sym.CPMQDNAL.newTable  ExtrapMethod=Clip  InternalRulePriority=Speed  RndMeth=Simplest  InputSameDT=on
      settings: InputPortMap=u0,u1
  Product1 : Product
  Product2 : Product
  Sum : Sum  Inputs=++|
  Sum1 : Sum  Inputs=|++
  mach_nd_cnst : Constant  Value=0.5
  Out1 : Outport
  wires:
  dN/1 -> CPMQDNAL_DN_ALFA/2
  tfhigh/1 -> Product2/2
  Sum1/1 -> Out1/1
  tflow/1 -> Product1/1
  angleOfAttack_deg/1 -> CPMQAM_ALFA_M/2, CPMQDNAL_DN_ALFA/1, CPMQAL_ALFA/1
  Product2/1 -> Sum1/2
  CPMQAM_ALFA_M/1 -> Product2/1
  CPMQAL_ALFA/1 -> Sum/1
  mach_nd_cnst/1 -> CPMQAM_ALFA_M/1
  Sum/1 -> Product1/2
  Product1/1 -> Sum1/1
  CPMQDNAL_DN_ALFA/1 -> Sum/2

== system aerotest/PitchMomentCoefficient/MachRegion3/Cpmdei/Subsystem ==
  dEI : Inport
  angleOfAttack_deg : Inport  Port=2
  eieff : Inport  Port=3
  mach_nd : Inport  Port=4
  CPMMDEA_ALFA_DE_M : Lookup_n-D  NumberOfTableDimensions=3  BreakpointsForDimension1=admireDB.aerodata_sym.CPMMDEA.breakpoints.ALFA  BreakpointsForDimension2=admireDB.aerodata_sym.CPMMDEA.breakpoints.DE  BreakpointsForDimension3=admireDB.aerodata_sym.CPMMDEA.breakpoints.M  Table=admireDB.aerodata_sym.CPMMDEA.newTable  ExtrapMethod=Clip  InternalRulePriority=Speed  RndMeth=Simplest  InputSameDT=on
      settings: InputPortMap=u0,u1,u2
  CPMMDEA_ALFA_DE_M1 : Lookup_n-D  NumberOfTableDimensions=3  BreakpointsForDimension1=admireDB.aerodata_sym.CPMMDEA.breakpoints.ALFA  BreakpointsForDimension2=admireDB.aerodata_sym.CPMMDEA.breakpoints.DE  BreakpointsForDimension3=admireDB.aerodata_sym.CPMMDEA.breakpoints.M  Table=admireDB.aerodata_sym.CPMMDEA.newTable  ExtrapMethod=Clip  InternalRulePriority=Speed  RndMeth=Simplest  InputSameDT=on
      settings: InputPortMap=u0,u1,u2
  Constant : Constant  Value=0
  Product : Product
  Sum : Sum  Inputs=|+-
  Out1 : Outport
  wires:
  Constant/1 -> CPMMDEA_ALFA_DE_M1/2
  mach_nd/1 -> CPMMDEA_ALFA_DE_M1/3, CPMMDEA_ALFA_DE_M/3
  eieff/1 -> Product/2
  angleOfAttack_deg/1 -> CPMMDEA_ALFA_DE_M/1, CPMMDEA_ALFA_DE_M1/1
  Sum/1 -> Product/1
  CPMMDEA_ALFA_DE_M1/1 -> Sum/2
  CPMMDEA_ALFA_DE_M/1 -> Sum/1
  Product/1 -> Out1/1
  dEI/1 -> CPMMDEA_ALFA_DE_M/2

== system aerotest/PitchMomentCoefficient/MachRegion3/Cpmdey/Subsystem ==
  dEY : Inport
  angleOfAttack_deg : Inport  Port=2
  eoeff : Inport  Port=3
  mach_nd : Inport  Port=4
  CPMMDEA_ALFA_DE_M : Lookup_n-D  NumberOfTableDimensions=3  BreakpointsForDimension1=admireDB.aerodata_sym.CPMMDEA.breakpoints.ALFA  BreakpointsForDimension2=admireDB.aerodata_sym.CPMMDEA.breakpoints.DE  BreakpointsForDimension3=admireDB.aerodata_sym.CPMMDEA.breakpoints.M  Table=admireDB.aerodata_sym.CPMMDEA.newTable  ExtrapMethod=Clip  InternalRulePriority=Speed  RndMeth=Simplest  InputSameDT=on
      settings: InputPortMap=u0,u1,u2
  CPMMDEA_ALFA_DE_M1 : Lookup_n-D  NumberOfTableDimensions=3  BreakpointsForDimension1=admireDB.aerodata_sym.CPMMDEA.breakpoints.ALFA  BreakpointsForDimension2=admireDB.aerodata_sym.CPMMDEA.breakpoints.DE  BreakpointsForDimension3=admireDB.aerodata_sym.CPMMDEA.breakpoints.M  Table=admireDB.aerodata_sym.CPMMDEA.newTable  ExtrapMethod=Clip  InternalRulePriority=Speed  RndMeth=Simplest  InputSameDT=on
      settings: InputPortMap=u0,u1,u2
  Constant : Constant  Value=0
  Product : Product
  Sum : Sum  Inputs=|+-
  Out1 : Outport
  wires:
  dEY/1 -> CPMMDEA_ALFA_DE_M/2
  Product/1 -> Out1/1
  CPMMDEA_ALFA_DE_M/1 -> Sum/1
  CPMMDEA_ALFA_DE_M1/1 -> Sum/2
  Sum/1 -> Product/1
  angleOfAttack_deg/1 -> CPMMDEA_ALFA_DE_M1/1, CPMMDEA_ALFA_DE_M/1
  eoeff/1 -> Product/2
  mach_nd/1 -> CPMMDEA_ALFA_DE_M/3, CPMMDEA_ALFA_DE_M1/3
  Constant/1 -> CPMMDEA_ALFA_DE_M1/2

== system aerotest/PitchMomentCoefficient/MachRegion3/Cpmdle/Subsystem1 ==
  <qacorr> : Inport
  <mach_nd> : Inport  Port=2
  CPMEDLEI_QA_M : Lookup_n-D  BreakpointsForDimension1=admireDB.aerodata_sym.CPMEDLEI.breakpoints.M  BreakpointsForDimension2=admireDB.aerodata_sym.CPMEDLEI.breakpoints.QA  BreakpointsForDimension3=[5, 7]  Table=admireDB.aerodata_sym.CPMEDLEI.newTable  ExtrapMethod=Clip  InternalRulePriority=Speed  RndMeth=Simplest  InputSameDT=on
      settings: InputPortMap=u0,u1
  CPMEDLEY_QA_M : Lookup_n-D  BreakpointsForDimension1=admireDB.aerodata_sym.CPMEDLEY.breakpoints.M  BreakpointsForDimension2=admireDB.aerodata_sym.CPMEDLEY.breakpoints.QA  BreakpointsForDimension3=[5, 7]  Table=admireDB.aerodata_sym.CPMEDLEY.newTable  ExtrapMethod=Clip  InternalRulePriority=Speed  RndMeth=Simplest  InputSameDT=on
      settings: InputPortMap=u0,u1
  Sum1 : Sum  Inputs=|++
  Out1 : Outport
  wires:
  <mach_nd>/1 -> CPMEDLEY_QA_M/1, CPMEDLEI_QA_M/1
  CPMEDLEY_QA_M/1 -> Sum1/2
  CPMEDLEI_QA_M/1 -> Sum1/1
  <qacorr>/1 -> CPMEDLEY_QA_M/2, CPMEDLEI_QA_M/2
  Sum1/1 -> Out1/1

== system aerotest/RollMomentCoefficient/MachRegion1/Crmbasic/Crmbasic_ ==
  angleOfAttack_deg : Inport
  Abs : Abs
  CRMZERO_ALFA : Lookup_n-D  NumberOfTableDimensions=1  BreakpointsForDimension1=admireDB.aerodata_asym_ext.CRMZERO.breakpoints.ALFA  BreakpointsForDimension3=[5, 7]  Table=admireDB.aerodata_asym_ext.CRMZERO.newTable  ExtrapMethod=Clip  InternalRulePriority=Speed  RndMeth=Simplest  InputSameDT=on
  Crmbasic : Outport
  wires:
  Abs/1 -> CRMZERO_ALFA/1
  angleOfAttack_deg/1 -> Abs/1
  CRMZERO_ALFA/1 -> Crmbasic/1

== system aerotest/RollMomentCoefficient/MachRegion1/Crmbde/Crmbde_ ==
  angleOfAttack_deg : Inport
  dN : Inport  Port=2
  dEI : Inport  Port=3
  angleOfSideslip_deg : Inport  Port=4
  dEY : Inport  Port=5
  eieff : Inport  Port=6
  eoeff : Inport  Port=7
  Abs : Abs
  CRMDEB_ALFA_DN_DE_BETA : Lookup_n-D  NumberOfTableDimensions=4  BreakpointsForDimension1=admireDB.aerodata_asym_ext.CRMDEB.breakpoints.ALFA  BreakpointsForDimension2=admireDB.aerodata_asym_ext.CRMDEB.breakpoints.DN  BreakpointsForDimension3=admireDB.aerodata_asym_ext.CRMDEB.breakpoints.DE  BreakpointsForDimension4=admireDB.aerodata_asym_ext.CRMDEB.breakpoints.BETA  Table=admireDB.aerodata_asym_ext.CRMDEB.newTable  ExtrapMethod=Clip  InternalRulePriority=Speed  RndMeth=Simplest  InputSameDT=on
      settings: InputPortMap=u0,u1,u2,u3
  CRMDEB_ALFA_DN_DE_BETA_1 : Lookup_n-D  NumberOfTableDimensions=4  BreakpointsForDimension1=admireDB.aerodata_asym_ext.CRMDEB.breakpoints.ALFA  BreakpointsForDimension2=admireDB.aerodata_asym_ext.CRMDEB.breakpoints.DN  BreakpointsForDimension3=admireDB.aerodata_asym_ext.CRMDEB.breakpoints.DE  BreakpointsForDimension4=admireDB.aerodata_asym_ext.CRMDEB.breakpoints.BETA  Table=admireDB.aerodata_asym_ext.CRMDEB.newTable  ExtrapMethod=Clip  InternalRulePriority=Speed  RndMeth=Simplest  InputSameDT=on
      settings: InputPortMap=u0,u1,u2,u3
  Product : Product  Inputs=**
  Product1 : Product  Inputs=**
  Product2 : Product
  Sign : Signum
  Sum : Sum  Inputs=|++
  Crmbde : Outport
  wires:
  dEY/1 -> CRMDEB_ALFA_DN_DE_BETA_1/3
  dEI/1 -> CRMDEB_ALFA_DN_DE_BETA/3
  dN/1 -> CRMDEB_ALFA_DN_DE_BETA_1/2, CRMDEB_ALFA_DN_DE_BETA/2
  angleOfAttack_deg/1 -> CRMDEB_ALFA_DN_DE_BETA_1/1, CRMDEB_ALFA_DN_DE_BETA/1
  Sign/1 -> Product2/1
  Product2/1 -> Crmbde/1
  Product1/1 -> Sum/2
  Product/1 -> Sum/1
  Sum/1 -> Product2/2
  eoeff/1 -> Product1/1
  eieff/1 -> Product/2
  CRMDEB_ALFA_DN_DE_BETA_1/1 -> Product1/2
  CRMDEB_ALFA_DN_DE_BETA/1 -> Product/1
  Abs/1 -> CRMDEB_ALFA_DN_DE_BETA_1/4, CRMDEB_ALFA_DN_DE_BETA/4
  angleOfSideslip_deg/1 -> Abs/1, Sign/1

== system aerotest/RollMomentCoefficient/MachRegion1/Crmbdle/Crmbdle_ ==
  dLE : Inport
  angleOfSideslip_deg : Inport  Port=2
  dEI : Inport  Port=3
  angleOfAttack_deg : Inport  Port=4
  dEY : Inport  Port=5
  eieff : Inport  Port=6
  eoeff : Inport  Port=7
  Abs : Abs
  CRMDLEB_ALFA_DE_BETA_DLE : Lookup_n-D  NumberOfTableDimensions=4  BreakpointsForDimension1=admireDB.aerodata_asym_ext.CRMDLEB.breakpoints.ALFA  BreakpointsForDimension2=admireDB.aerodata_asym_ext.CRMDLEB.breakpoints.DE  BreakpointsForDimension3=admireDB.aerodata_asym_ext.CRMDLEB.breakpoints.BETA  BreakpointsForDimension4=admireDB.aerodata_asym_ext.CRMDLEB.breakpoints.DLE  Table=admireDB.aerodata_asym_ext.CRMDLEB.newTable  ExtrapMethod=Clip  InternalRulePriority=Speed  RndMeth=Simplest  InputSameDT=on
      settings: InputPortMap=u0,u1,u2,u3
  CRMDLEB_ALFA_DE_BETA_DLE_1 : Lookup_n-D  NumberOfTableDimensions=4  BreakpointsForDimension1=admireDB.aerodata_asym_ext.CRMDLEB.breakpoints.ALFA  BreakpointsForDimension2=admireDB.aerodata_asym_ext.CRMDLEB.breakpoints.DE  BreakpointsForDimension3=admireDB.aerodata_asym_ext.CRMDLEB.breakpoints.BETA  BreakpointsForDimension4=admireDB.aerodata_asym_ext.CRMDLEB.breakpoints.DLE  Table=admireDB.aerodata_asym_ext.CRMDLEB.newTable  ExtrapMethod=Clip  InternalRulePriority=Speed  RndMeth=Simplest  InputSameDT=on
      settings: InputPortMap=u0,u1,u2,u3
  Product1 : Product  Inputs=**
  Product2 : Product  Inputs=**
  Product3 : Product
  Sign : Signum
  Sum : Sum  Inputs=|++
  Crmbdle : Outport
  wires:
  dEY/1 -> CRMDLEB_ALFA_DE_BETA_DLE_1/2
  dEI/1 -> CRMDLEB_ALFA_DE_BETA_DLE/2
  Abs/1 -> CRMDLEB_ALFA_DE_BETA_DLE_1/3, CRMDLEB_ALFA_DE_BETA_DLE/3
  dLE/1 -> CRMDLEB_ALFA_DE_BETA_DLE_1/4, CRMDLEB_ALFA_DE_BETA_DLE/4
  CRMDLEB_ALFA_DE_BETA_DLE/1 -> Product1/1
  eoeff/1 -> Product2/1
  Product1/1 -> Sum/1
  Sum/1 -> Product3/2
  CRMDLEB_ALFA_DE_BETA_DLE_1/1 -> Product2/2
  Sign/1 -> Product3/1
  eieff/1 -> Product1/2
  Product2/1 -> Sum/2
  angleOfSideslip_deg/1 -> Abs/1, Sign/1
  angleOfAttack_deg/1 -> CRMDLEB_ALFA_DE_BETA_DLE_1/1, CRMDLEB_ALFA_DE_BETA_DLE/1
  Product3/1 -> Crmbdle/1

== system aerotest/RollMomentCoefficient/MachRegion1/Crmbdn/Crmbdn_ ==
  angleOfAttack_deg : Inport
  dN : Inport  Port=2
  angleOfSideslip_deg : Inport  Port=3
  Abs : Abs
  CRMDNB_ALFA_DN_BETA : Lookup_n-D  NumberOfTableDimensions=3  BreakpointsForDimension1=admireDB.aerodata_asym_ext.CRMDNB.breakpoints.ALFA  BreakpointsForDimension2=admireDB.aerodata_asym_ext.CRMDNB.breakpoints.DN  BreakpointsForDimension3=admireDB.aerodata_asym_ext.CRMDNB.breakpoints.BETA  Table=admireDB.aerodata_asym_ext.CRMDNB.newTable  ExtrapMethod=Clip  InternalRulePriority=Speed  RndMeth=Simplest  InputSameDT=on
      settings: InputPortMap=u0,u1,u2
  Product : Product
  Sign : Signum
  Crmbdn : Outport
  wires:
  Sign/1 -> Product/2
  CRMDNB_ALFA_DN_BETA/1 -> Product/1
  angleOfSideslip_deg/1 -> Abs/1, Sign/1
  angleOfAttack_deg/1 -> CRMDNB_ALFA_DN_BETA/1
  dN/1 -> CRMDNB_ALFA_DN_BETA/2
  Abs/1 -> CRMDNB_ALFA_DN_BETA/3
  Product/1 -> Crmbdn/1
